simulink model "power_transfo3wdn"  (Simulink 6.0)
settings: Solver=ode15s  StartTime=0.0  StopTime=0.5  RelTol=1e-3
undefined symbols (not defined in the file or in its folder): D1, Delta
libraries: powerlib x28
settings Model: Creator=patrice  LastModifiedBy=batserve  ExtModeTrigMode=oneshot  ExtModeArmWhenConnect=off  ExtModeAutoUpdateStatusClock=off
settings DataIOCC: LimitDataPoints=off  SignalLoggingName=sigsOut
settings OptimizationCC: BooleanDataType=off
settings DebuggingCC: SolverPrmCheckMsg=none
settings HardwareCC: TargetUnknown=on

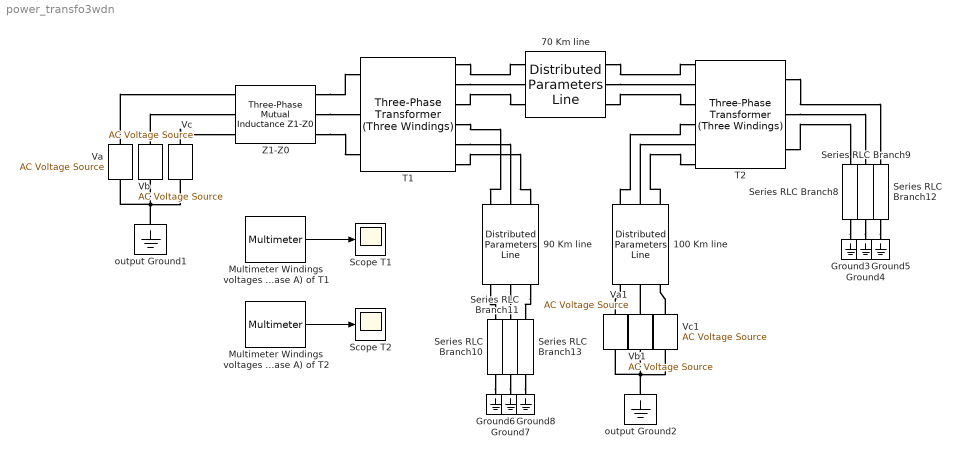
== system power_transfo3wdn ==
  100 Km line : powerlib/Elements/Distributed Parameters Line  Orientation=up  Phases=3  Frequency=60  Resistance=[0.045 0.383]  Inductance="[0.0009536  .0034]"  Capacitance="[12.02e-9   7.47e-9]"  Length=100  x1=[0 0.7635 6.552e+04 -3.356e+05;0.0004716 0.2984 1.238e+05 -3.187e+05;0.0009433 -0.1761 1.782e+05 -2.918e+05;0.001415 -0.645 2.27e+05 -2.556e+05;0.001887 -1.094 2.687e+05 -2.114e+05;0.002358 -1.508 3.018e+05 -1.606e+05]  x2=[0 1.583 2.165e+04 -3.402e+05;0.0004716 0.789 8.149e+04 -3.31e+05;0.0009433 -0.02989 1.388e+05 -3.114e+05;0.001415 -0.8479 1.916e+05 -2.82e+05;0.001887 -1.639 2.385e+05 -2.436e+05;0.002358 -2.379 2.778e+05 -1.976e+05]  x3=[0 0.02395 -235.2 649.9;0.0004716 0.02363 -346.5 598;0.0009433 0.02255 -446.8 527.3;0.001415 0.02077 -533 440;0.001887 0.01833 -602.4 338.8;0.002358 0.01531 -652.8 226.9]  x4=[0 -0.01995 443.3 -3029;0.0004716 -0.02141 972 -2902;0.0009433 -0.02221 1470 -2685;0.001415 -0.0223 1922 -2382;0.001887 -0.02169 2313 -2005;0.002358 -0.02039 2631 -1564]  x5=0.002358  Measurements=None
      settings: AttributesFormatString=\n
  70 Km line : powerlib/Elements/Distributed Parameters Line  Phases=3  Frequency=60  Resistance=[0.045 0.383]  Inductance="[0.0009536  .0034]"  Capacitance="[12.02e-9   7.47e-9]"  Length=70  x1=[0 0.7635 6.552e+04 -3.356e+05;0.0004716 0.2984 1.238e+05 -3.187e+05;0.0009433 -0.1761 1.782e+05 -2.918e+05;0.001415 -0.645 2.27e+05 -2.556e+05;0.001887 -1.094 2.687e+05 -2.114e+05;0.002358 -1.508 3.018e+05 -1.606e+05]  x2=[0 1.583 2.165e+04 -3.402e+05;0.0004716 0.789 8.149e+04 -3.31e+05;0.0009433 -0.02989 1.388e+05 -3.114e+05;0.001415 -0.8479 1.916e+05 -2.82e+05;0.001887 -1.639 2.385e+05 -2.436e+05;0.002358 -2.379 2.778e+05 -1.976e+05]  x3=[0 0.02395 -235.2 649.9;0.0004716 0.02363 -346.5 598;0.0009433 0.02255 -446.8 527.3;0.001415 0.02077 -533 440;0.001887 0.01833 -602.4 338.8;0.002358 0.01531 -652.8 226.9]  x4=[0 -0.01995 443.3 -3029;0.0004716 -0.02141 972 -2902;0.0009433 -0.02221 1470 -2685;0.001415 -0.0223 1922 -2382;0.001887 -0.02169 2313 -2005;0.002358 -0.02039 2631 -1564]  x5=0.002358  Measurements=None
      settings: AttributesFormatString=\n
  90 Km line : powerlib/Elements/Distributed Parameters Line  Orientation=down  Phases=3  Frequency=60  Resistance=[0.045 0.383]  Inductance="[0.0009536  .0034]"  Capacitance="[12.02e-9   7.47e-9]"  Length=90  x1=[0 0.7635 6.552e+04 -3.356e+05;0.0004716 0.2984 1.238e+05 -3.187e+05;0.0009433 -0.1761 1.782e+05 -2.918e+05;0.001415 -0.645 2.27e+05 -2.556e+05;0.001887 -1.094 2.687e+05 -2.114e+05;0.002358 -1.508 3.018e+05 -1.606e+05]  x2=[0 1.583 2.165e+04 -3.402e+05;0.0004716 0.789 8.149e+04 -3.31e+05;0.0009433 -0.02989 1.388e+05 -3.114e+05;0.001415 -0.8479 1.916e+05 -2.82e+05;0.001887 -1.639 2.385e+05 -2.436e+05;0.002358 -2.379 2.778e+05 -1.976e+05]  x3=[0 0.02395 -235.2 649.9;0.0004716 0.02363 -346.5 598;0.0009433 0.02255 -446.8 527.3;0.001415 0.02077 -533 440;0.001887 0.01833 -602.4 338.8;0.002358 0.01531 -652.8 226.9]  x4=[0 -0.01995 443.3 -3029;0.0004716 -0.02141 972 -2902;0.0009433 -0.02221 1470 -2685;0.001415 -0.0223 1922 -2382;0.001887 -0.02169 2313 -2005;0.002358 -0.02039 2631 -1564]  x5=0.002358  Measurements=None
      settings: AttributesFormatString=\n
  Ground{3..8} (6 alike) : powerlib/Elements/Ground  Orientation=down  PhysicalDomain=powersysdomain  SubClassName=unknown  LeftPortType=p1  RightPortType=p1  LConnTagsString=a
  Multimeter Windings voltages (phase A) of T1 : powerlib/Measurements/Multimeter  Tag=PoWeRsYsTeMmEaSuReMeNt  PhasorSimulation=off  OutputType=Magnitude  sel=[1 4 7]  L=18  Gain=[1 1 1]  yselected={'Uag_w1: T1','Uag_w2: T1','Uab_w3: T1'};  PSBOutputType=1  PSBequivalent=0  AxesSetting=[0,0.1,-100,100]  Display=0  SavedBlockNames={}
      settings: AttributesFormatString=\n
  Multimeter Windings voltages (phase A) of T2 : powerlib/Measurements/Multimeter  Tag=PoWeRsYsTeMmEaSuReMeNt  PhasorSimulation=off  OutputType=Magnitude  sel=[10 13 16]  L=18  Gain=[1 1 1]  yselected={'Uan_w1: T2','Uan_w2: T2','Uab_w3: T2'};  PSBOutputType=1  PSBequivalent=0  AxesSetting=[0,0.1,-100,100]  Display=0  SavedBlockNames={}
      settings: AttributesFormatString=\n
  Scope T1 : Scope
      settings: TimeRange=0.1  YMin=-400000  YMax=400000
  Scope T2 : Scope
      settings: TimeRange=0.1  YMin=-1e+006  YMax=1e+006
  Series RLC Branch{8..13} (6 alike) : powerlib/Elements/Series RLC Branch  Orientation=down  PhysicalDomain=powersysdomain  SubClassName=unknown  LeftPortType=p1  RightPortType=p1  LConnTagsString=__new0  RConnTagsString=__new0  Resistance=5.7  Inductance=6.03  Capacitance=inf  Measurements=None
  T1 : powerlib/Elements/Three-Phase Transformer (Three Windings)  NominalPower=[ 250e6 , 60 ]  Winding1Connection=Yg  Winding1=[ 735e3 , 0.002 , 0.08 ]  Winding2Connection=Yg  Winding2=[ 315e3 , 0.002 , 0.08 ]  Winding3Connection=Delta (D1)  Winding3=[ 315e3 , 0.002 , 0.08 ]  SetSaturation=off  Rm=500  Lm=500  Saturation="[ 0,0  ;  0.005,1.2  ;  1.0,1.4]"  Hysteresis=off  DataFile='hysteresis'  SetInitialFlux=off  InitialFluxes=[0.8 -0.8 0.7]  Measurements=Winding voltages  TransfoNumber=0
      settings: AttributesFormatString=\n
  T2 : powerlib/Elements/Three-Phase Transformer (Three Windings)  Orientation=left  NominalPower=[ 250e6 , 60 ]  Winding1Connection=Y  Winding1=[ 735e3 , 0.002 , 0.08 ]  Winding2Connection=Y  Winding2=[ 315e3 , 0.002 , 0.08 ]  Winding3Connection=Delta (D1)  Winding3=[ 315e3 , 0.002 , 0.08 ]  SetSaturation=off  Rm=500  Lm=500  Saturation="[ 0,0  ;  0.005,1.2  ;  1.0,1.4]"  Hysteresis=off  DataFile='hysteresis'  SetInitialFlux=off  InitialFluxes=[0.8 -0.8 0.7]  Measurements=Winding voltages  TransfoNumber=0
      settings: AttributesFormatString=\n
  Va : powerlib/Electrical Sources/AC Voltage Source  Description=source block  Orientation=up  Amplitude=315e3  Phase=-65.4  Frequency=60  SampleTime=0  Measurements=None
      settings: AttributesFormatString=\n
  Va1 : powerlib/Electrical Sources/AC Voltage Source  Description=source block  Orientation=up  Amplitude=479690  Phase=0  Frequency=60  SampleTime=0  Measurements=None
      settings: AttributesFormatString=\n
  Vb : powerlib/Electrical Sources/AC Voltage Source  Description=source block  Orientation=up  Amplitude=315e3  Phase=-65.4-120  Frequency=60  SampleTime=0  Measurements=None
      settings: AttributesFormatString=\n
  Vb1 : powerlib/Electrical Sources/AC Voltage Source  Description=source block  Orientation=up  Amplitude=470000  Phase=-120  Frequency=60  SampleTime=0  Measurements=None
      settings: AttributesFormatString=\n
  Vc : powerlib/Electrical Sources/AC Voltage Source  Description=source block  Orientation=up  Amplitude=479690  Phase=-65.4+120  Frequency=60  SampleTime=0  Measurements=None
      settings: AttributesFormatString=\n
  Vc1 : powerlib/Electrical Sources/AC Voltage Source  Description=source block  Orientation=up  Amplitude=470000  Phase=+120  Frequency=60  SampleTime=0  Measurements=None
      settings: AttributesFormatString=\n
  Z1-Z0 : powerlib/Elements/Three-Phase Mutual Inductance Z1-Z0  PhysicalDomain=powersysdomain  SubClassName=unknown  LeftPortType=p1  RightPortType=p1  LConnTagsString=a|b|c  RConnTagsString=A|B|C  PositiveSequence="[ 2  50e-3]"  ZeroSequence="[4  100e-3]"
  output Ground1 : powerlib/Elements/Ground  Orientation=down  PhysicalDomain=powersysdomain  SubClassName=unknown  LeftPortType=p1  RightPortType=p1  LConnTagsString=a
  output Ground2 : powerlib/Elements/Ground  Orientation=down  PhysicalDomain=powersysdomain  SubClassName=unknown  LeftPortType=p1  RightPortType=p1  LConnTagsString=a
  wires:
  Multimeter Windings voltages (phase A) of T1/1 -> Scope T1/1
  Multimeter Windings voltages (phase A) of T2/1 -> Scope T2/1
  connections:
  T1/RConn2 -- 70 Km line/LConn2
  T1/RConn3 -- 70 Km line/LConn3
  T1/RConn1 -- 70 Km line/LConn1
  T2/LConn3 -- Series RLC Branch8/LConn1
  T2/LConn2 -- Series RLC Branch9/LConn1
  T2/LConn1 -- Series RLC Branch12/LConn1
  70 Km line/RConn2 -- T2/RConn2
  70 Km line/RConn1 -- T2/RConn1
  70 Km line/RConn3 -- T2/RConn3
  Series RLC Branch8/RConn1 -- Ground3/LConn1
  Series RLC Branch9/RConn1 -- Ground4/LConn1
  Series RLC Branch12/RConn1 -- Ground5/LConn1
  T1/RConn4 -- 90 Km line/LConn1
  T1/RConn5 -- 90 Km line/LConn2
  T1/RConn6 -- 90 Km line/LConn3
  Z1-Z0/RConn1 -- T1/LConn1
  Z1-Z0/RConn2 -- T1/LConn2
  Z1-Z0/RConn3 -- T1/LConn3
  Vc/RConn1 -- Z1-Z0/LConn3
  Vb/RConn1 -- Z1-Z0/LConn2
  Va/RConn1 -- Z1-Z0/LConn1
  output Ground1/LConn1 -- Vc/LConn1 -- Va/LConn1 -- Vb/LConn1
  Series RLC Branch10/RConn1 -- Ground6/LConn1
  Series RLC Branch11/RConn1 -- Ground7/LConn1
  Series RLC Branch13/RConn1 -- Ground8/LConn1
  90 Km line/RConn2 -- Series RLC Branch11/LConn1
  90 Km line/RConn3 -- Series RLC Branch13/LConn1
  90 Km line/RConn1 -- Series RLC Branch10/LConn1
  100 Km line/RConn3 -- T2/RConn6
  100 Km line/RConn2 -- T2/RConn5
  100 Km line/RConn1 -- T2/RConn4
  output Ground2/LConn1 -- Vb1/LConn1 -- Va1/LConn1 -- Vc1/LConn1
  Vb1/RConn1 -- 100 Km line/LConn2
  Va1/RConn1 -- 100 Km line/LConn1
  Vc1/RConn1 -- 100 Km line/LConn3
